simulink model "Problem4_Simulink_Diagram"  (R2025b)
settings: Solver=ode45  StartTime=0.0  StopTime=24  MaxStep=0.1  RelTol=1e-3
undefined symbols (not defined in the file or in its folder): sigbuilder_block
settings Model: Creator=Rashid  LastModifiedBy=Rashid

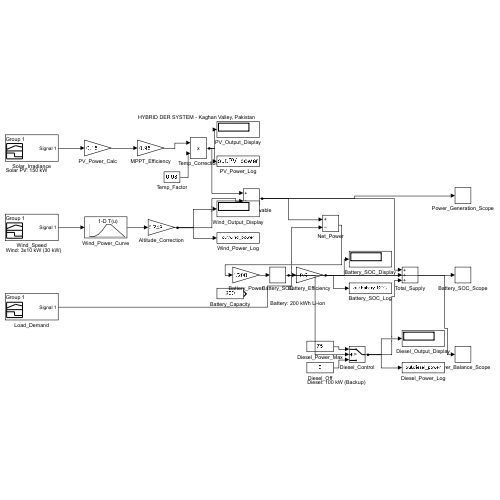
[thumbnail: Simulink's stored preview of the top-level diagram]
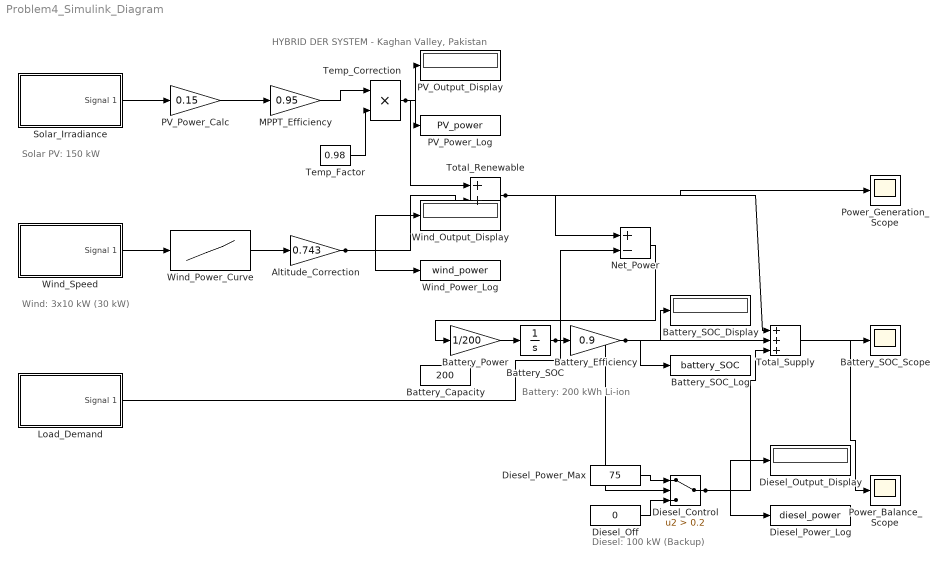
== system Problem4_Simulink_Diagram ==
  note: HYBRID DER SYSTEM - Kaghan Valley, Pakistan
  note: Solar PV: 150 kW
  note: Wind: 3x10 kW (30 kW)
  note: Battery: 200 kWh Li-ion
  note: Diesel: 100 kW (Backup)
  Altitude_Correction : Gain  Gain=0.743
  Battery_Capacity : Constant  Value=200
  Battery_Efficiency : Gain  Gain=0.9
  Battery_Power : Gain  Gain=1/200
  Battery_SOC : Integrator  InitialCondition=0.5  UpperSaturationLimit=1.0  LowerSaturationLimit=0.0
  Battery_SOC_Display : Display
  Battery_SOC_Log : ToWorkspace  VariableName=battery_SOC  SaveFormat=Timeseries  SampleTime=-1
  Battery_SOC_Scope : Scope
  Diesel_Control : Switch  Criteria=u2 > Threshold  Threshold=0.2  SaturateOnIntegerOverflow=off  InputSameDT=off
  Diesel_Off : Constant  Value=0
  Diesel_Output_Display : Display
  Diesel_Power_Log : ToWorkspace  VariableName=diesel_power  SaveFormat=Timeseries  SampleTime=-1
  Diesel_Power_Max : Constant  Value=75
  Load_Demand : Subsystem  Tag=STV Subsys  LoadFcn=sigbuilder_block('load');  StartFcn=sigbuilder_block('start');  StopFcn=sigbuilder_block('stop');  ClipboardFcn=sigbuilder_block('clipboard');  mask(Sigbuilder block){tuvar=[0:10]}
      mask help: Simulink:masks:SigbuilderBlock_MD
      mask init:
      | if ~strcmp(get_param(bdroot(gcbh),'SimulationStatus'),'stopped') tuvar = sigbuilder_block('maskInit'); end
      settings: CopyFcn=sigbuilder_block('copy');  DeleteFcn=sigbuilder_block('delete');  ModelCloseFcn=sigbuilder_block('modelClose');  PreSaveFcn=sigbuilder_block('preSave');  PauseFcn=sigbuilder_block('pause');  ContinueFcn=sigbuilder_block('continue');  NameChangeFcn=sigbuilder_block('namechange');  OpenFcn=sigbuilder_block('open',[437.6 199.2 550.4 400 ]);  CloseFcn=sigbuilder_block('close');
      mask Display: plot(0, 0, 100, 100,[2, 2, 32, 32, 2], [68, 8, 8, 68, 68],[32, 2], [38, 38], [32, 19, 2],[53, 60, 44], [32, 17, 17, 2],[16, 16, 31, 31]);txt = getActiveGroup(gcbh);text(2, 100, txt,'verticalAlignment', 'top');
  MPPT_Efficiency : Gain  Gain=0.95
  Net_Power : Sum  Inputs=+-
  PV_Output_Display : Display
  PV_Power_Calc : Gain  Gain=0.15
  PV_Power_Log : ToWorkspace  VariableName=PV_power  SaveFormat=Timeseries  SampleTime=-1
  Power_Balance_Scope : Scope
  Power_Generation_Scope : Scope
  Solar_Irradiance : Subsystem  Tag=STV Subsys  LoadFcn=sigbuilder_block('load');  StartFcn=sigbuilder_block('start');  StopFcn=sigbuilder_block('stop');  ClipboardFcn=sigbuilder_block('clipboard');  mask(Sigbuilder block){tuvar=[0:10]}
      mask help: Simulink:masks:SigbuilderBlock_MD
      mask init:
      | if ~strcmp(get_param(bdroot(gcbh),'SimulationStatus'),'stopped') tuvar = sigbuilder_block('maskInit'); end
      settings: CopyFcn=sigbuilder_block('copy');  DeleteFcn=sigbuilder_block('delete');  ModelCloseFcn=sigbuilder_block('modelClose');  PreSaveFcn=sigbuilder_block('preSave');  PauseFcn=sigbuilder_block('pause');  ContinueFcn=sigbuilder_block('continue');  NameChangeFcn=sigbuilder_block('namechange');  OpenFcn=sigbuilder_block('open',[437.6 199.2 550.4 400 ]);  CloseFcn=sigbuilder_block('close');
      mask Display: plot(0, 0, 100, 100,[2, 2, 32, 32, 2], [68, 8, 8, 68, 68],[32, 2], [38, 38], [32, 19, 2],[53, 60, 44], [32, 17, 17, 2],[16, 16, 31, 31]);txt = getActiveGroup(gcbh);text(2, 100, txt,'verticalAlignment', 'top');
  Temp_Correction : Product
  Temp_Factor : Constant  Value=0.98
  Total_Renewable : Sum
  Total_Supply : Sum  Inputs=+++
  Wind_Output_Display : Display
  Wind_Power_Curve : Lookup_n-D  NumberOfTableDimensions=1  BreakpointsForDimension1=[0 3 6 9 12 15 25]  Table=[0 0 5 15 30 30 0]  InternalRulePriority=Speed  RndMeth=Simplest
  Wind_Power_Log : ToWorkspace  VariableName=wind_power  SaveFormat=Timeseries  SampleTime=-1
  Wind_Speed : Subsystem  Tag=STV Subsys  LoadFcn=sigbuilder_block('load');  StartFcn=sigbuilder_block('start');  StopFcn=sigbuilder_block('stop');  ClipboardFcn=sigbuilder_block('clipboard');  mask(Sigbuilder block){tuvar=[0:10]}
      mask help: Simulink:masks:SigbuilderBlock_MD
      mask init:
      | if ~strcmp(get_param(bdroot(gcbh),'SimulationStatus'),'stopped') tuvar = sigbuilder_block('maskInit'); end
      settings: CopyFcn=sigbuilder_block('copy');  DeleteFcn=sigbuilder_block('delete');  ModelCloseFcn=sigbuilder_block('modelClose');  PreSaveFcn=sigbuilder_block('preSave');  PauseFcn=sigbuilder_block('pause');  ContinueFcn=sigbuilder_block('continue');  NameChangeFcn=sigbuilder_block('namechange');  OpenFcn=sigbuilder_block('open',[437.6 199.2 550.4 400 ]);  CloseFcn=sigbuilder_block('close');
      mask Display: plot(0, 0, 100, 100,[2, 2, 32, 32, 2], [68, 8, 8, 68, 68],[32, 2], [38, 38], [32, 19, 2],[53, 60, 44], [32, 17, 17, 2],[16, 16, 31, 31]);txt = getActiveGroup(gcbh);text(2, 100, txt,'verticalAlignment', 'top');
  wires:
  Solar_Irradiance/1(Signal 1) -> PV_Power_Calc/1
  PV_Power_Calc/1 -> MPPT_Efficiency/1
  MPPT_Efficiency/1 -> Temp_Correction/1
  Temp_Factor/1 -> Temp_Correction/2
  Temp_Correction/1 -> Total_Renewable/1, PV_Output_Display/1, PV_Power_Log/1
  Wind_Speed/1(Signal 1) -> Wind_Power_Curve/1
  Wind_Power_Curve/1 -> Altitude_Correction/1
  Altitude_Correction/1 -> Total_Renewable/2, Wind_Output_Display/1, Wind_Power_Log/1
  Load_Demand/1(Signal 1) -> Net_Power/2
  Total_Renewable/1 -> Net_Power/1, Total_Supply/1, Power_Generation_Scope/1
  Net_Power/1 -> Battery_Power/1
  Battery_Power/1 -> Battery_SOC/1
  Battery_SOC/1 -> Battery_Efficiency/1, Battery_SOC_Scope/1, Diesel_Control/2
  Battery_Efficiency/1 -> Battery_SOC_Display/1, Battery_SOC_Log/1, Total_Supply/2
  Diesel_Power_Max/1 -> Diesel_Control/1
  Diesel_Off/1 -> Diesel_Control/3
  Diesel_Control/1 -> Diesel_Output_Display/1, Diesel_Power_Log/1, Total_Supply/3
  Total_Supply/1 -> Power_Balance_Scope/1

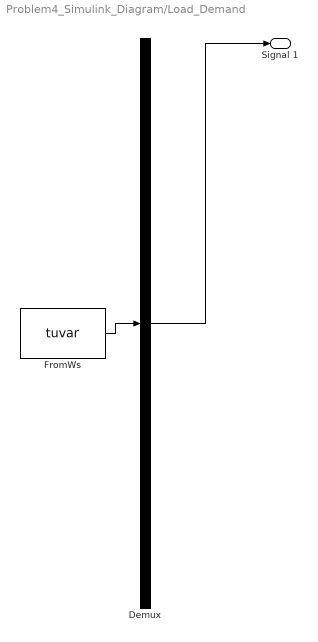
== system Problem4_Simulink_Diagram/Load_Demand ==
  Demux : Demux  Tag=STV Demux  Outputs=1
      settings: DisplayOption=none
  FromWs : FromWorkspace  Tag=STV FromWs  VariableName=tuvar
      SigBuilderData=|
      | common.afterFinalStr = 'Extrapolate'
      | common.sampleTime = 0
      | dataSet.timeRange = [0 10]
      | dataSet.name = 'Group 1'
      | sbobj.Groups.Name = 'Group 1'
      | sbobj.Groups.Signals.Name = 'Signal 1'
      | sbobj.Groups.Signals.XData = [0 4 4 6 6 10]
      | sbobj.Groups.Signals.YData = [0 0 1 1 0 0]
  Signal 1 : Outport  Tag=STV Outport
  wires:
  FromWs/1 -> Demux/1
  Demux/1 -> Signal 1/1

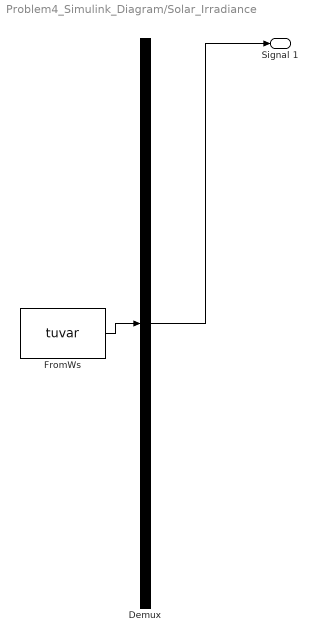
== system Problem4_Simulink_Diagram/Solar_Irradiance ==
  Demux : Demux  Tag=STV Demux  Outputs=1
      settings: DisplayOption=none
  FromWs : FromWorkspace  Tag=STV FromWs  VariableName=tuvar
      SigBuilderData=|
      | common.afterFinalStr = 'Extrapolate'
      | common.sampleTime = 0
      | dataSet.timeRange = [0 10]
      | dataSet.name = 'Group 1'
      | sbobj.Groups.Name = 'Group 1'
      | sbobj.Groups.Signals.Name = 'Signal 1'
      | sbobj.Groups.Signals.XData = [0 4 4 6 6 10]
      | sbobj.Groups.Signals.YData = [0 0 1 1 0 0]
  Signal 1 : Outport  Tag=STV Outport
  wires:
  FromWs/1 -> Demux/1
  Demux/1 -> Signal 1/1

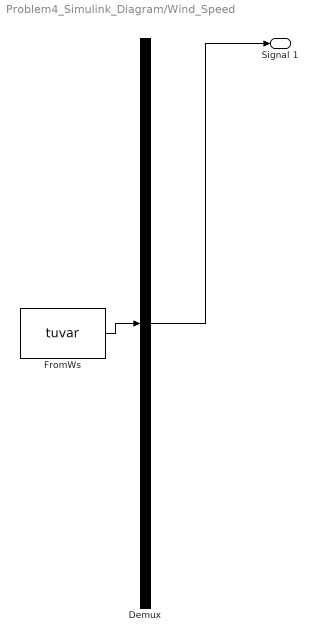
== system Problem4_Simulink_Diagram/Wind_Speed ==
  Demux : Demux  Tag=STV Demux  Outputs=1
      settings: DisplayOption=none
  FromWs : FromWorkspace  Tag=STV FromWs  VariableName=tuvar
      SigBuilderData=|
      | common.afterFinalStr = 'Extrapolate'
      | common.sampleTime = 0
      | dataSet.timeRange = [0 10]
      | dataSet.name = 'Group 1'
      | sbobj.Groups.Name = 'Group 1'
      | sbobj.Groups.Signals.Name = 'Signal 1'
      | sbobj.Groups.Signals.XData = [0 4 4 6 6 10]
      | sbobj.Groups.Signals.YData = [0 0 1 1 0 0]
  Signal 1 : Outport  Tag=STV Outport
  wires:
  FromWs/1 -> Demux/1
  Demux/1 -> Signal 1/1
